simulink model "feedback_plant2"  (R2016a)
settings: Solver=FixedStepAuto  StartTime=0.0  StopTime=inf  MaxStep=0.1  RelTol=1e-3
libraries: xpcnilib x4, slrtlib x2
settings Model: ModifiedByFormat=The MathWorks Inc.  Creator=The MathWorks, Inc.  LastModifiedBy=The MathWorks Inc.
settings SolverCC: EnableConcurrentExecution=on
settings DataIOCC: LimitDataPoints=on  SaveFormat=Array  SaveOutput=off  SignalLogging=off  DSMLogging=off  SaveTime=off
settings OptimizationCC: BlockReduction=off  DefaultParameterBehavior=Inlined  OptimizeBlockIOStorage=off  BufferReuse=off  GlobalBufferReuse=off  ExpressionFolding=off  ExpressionDepthLimit=2147483647  LocalBlockOutputs=off
settings DebuggingCC: UnderspecifiedInitializationDetection=Classic  MergeDetectMultiDrivingBlocksExec=none  SolverPrmCheckMsg=warning  FcnCallInpInsideContextMsg=EnableAllAsWarning  AllowSymbolicDim=off  StateNameClashWarn=warning
settings HardwareCC: ProdBitPerPointer=32  ProdLargestAtomicFloat=None  ProdWordSize=32  ProdLongLongMode=on  ProdHWDeviceType=Generic->32-bit x86 compatible
settings ModelReferenceCC: ModelReferenceNumInstancesAllowed=Single  ModelReferenceMinAlgLoopOccurrences=on  PropagateSignalLabelsOutOfModel=off
settings RTWCC: SystemTargetFile=slrt.tlc  TemplateMakefile=slrt_default_tmf  Description=Simulink Real-Time
settings CodeAppCC: MaxIdLength=50
settings ConfigComp: CovModelRefEnable=Off  CovSFcnEnable=off

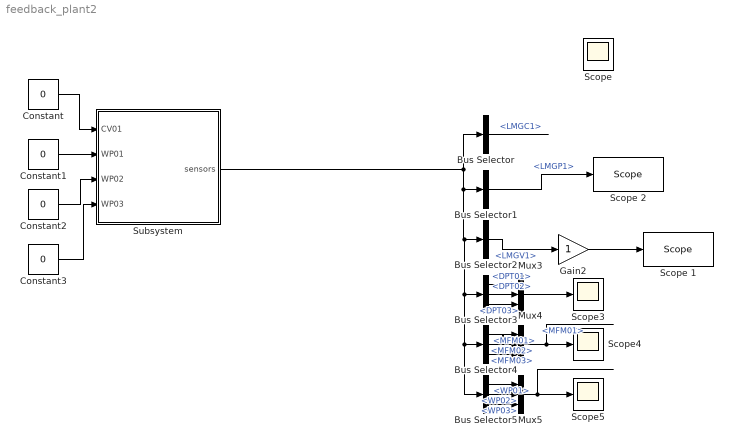
== system feedback_plant2 ==
  Bus Selector : BusSelector  OutputSignals=LMGC1
  Bus Selector1 : BusSelector  OutputSignals=LMGP1
  Bus Selector2 : BusSelector  OutputSignals=LMGV1
  Bus Selector3 : BusSelector  OutputSignals=DPT01,DPT02,DPT03
  Bus Selector4 : BusSelector  OutputSignals=MFM01,MFM02,MFM03
  Bus Selector5 : BusSelector  OutputSignals=WP01,WP02,WP03
  Constant{,1..3} (4 alike) : Constant  Value=0
  Gain2 : Gain
  Mux3 : Mux  Inputs=3
  Mux4 : Mux  Inputs=3
  Mux5 : Mux  Inputs=3
  Scope{,3..5} (4 alike) : Scope
  Scope 1 : slrtlib/Displays and Logging/Scope   scopeno=1  scopetype=Target  autostart=on  viewmode=Numerical  formatstr='%15.6f'  grid=on  ylimits=[0,0]  nosamples=250  noprepostsamples=0  interleave=1  triggermode=FreeRun  triggersignal=1  trigsignalfromport=off  triggerlevel=0.0  triggerslope=Either  triggerscope=1  triggersample=0  filename=data.dat  mode=Lazy  writesize=512  autorestart=off  dynamicfilemode=off  maxwritefilesize=512*1024^2
  Scope 2 : slrtlib/Displays and Logging/Scope   scopeno=2  scopetype=Target  autostart=on  viewmode=Numerical  formatstr='%15.6f'  grid=on  ylimits=[0,0]  nosamples=250  noprepostsamples=0  interleave=1  triggermode=FreeRun  triggersignal=1  trigsignalfromport=off  triggerlevel=0.0  triggerslope=Either  triggerscope=1  triggersample=0  filename=data.dat  mode=Lazy  writesize=512  autorestart=off  dynamicfilemode=off  maxwritefilesize=512*1024^2
  Subsystem : Subsystem
  wires:
  Mux3/1 -> Scope3/1
  Mux4/1 -> Scope4/1  "<MFM01>"
  Mux5/1 -> Scope5/1
  Constant/1 -> Subsystem/1(CV01)
  Constant1/1 -> Subsystem/2(WP01)
  Constant2/1 -> Subsystem/3(WP02)
  Constant3/1 -> Subsystem/4(WP03)
  Bus Selector3/1 -> Mux3/1  "<DPT01>"
  Bus Selector3/3 -> Mux3/3  "<DPT03>"
  Bus Selector3/2 -> Mux3/2  "<DPT02>"
  Bus Selector4/1 -> Mux4/1  "<MFM01>"
  Bus Selector4/3 -> Mux4/3  "<MFM03>"
  Bus Selector4/2 -> Mux4/2  "<MFM02>"
  Bus Selector5/1 -> Mux5/1  "<WP01>"
  Bus Selector5/2 -> Mux5/2  "<WP02>"
  Bus Selector5/3 -> Mux5/3  "<WP03>"
  Bus Selector/1 -> ?  "<LMGC1>"
  Subsystem/1(sensors) -> Bus Selector/1, Bus Selector5/1, Bus Selector4/1, Bus Selector3/1, Bus Selector2/1, Bus Selector1/1
  Bus Selector1/1 -> Scope 2/1  "<LMGP1>"
  Gain2/1 -> Scope 1/1
  Bus Selector2/1 -> Gain2/1  "<LMGV1>"

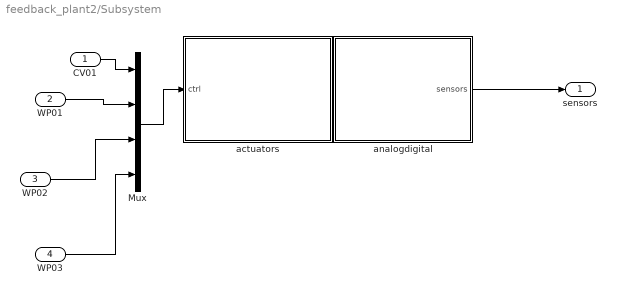
== system feedback_plant2/Subsystem ==
  CV01 : Inport
  WP01 : Inport  Port=2
  WP02 : Inport  Port=3
  WP03 : Inport  Port=4
  Mux : Mux
  actuators : Subsystem  mask{actuators_list={'CV03', 'CV05'}, subsystem=[3,1]}
      mask init:
      | %%Get analog channels
      | actuators = evalin('base','actuators');
      | 
      | subsystem = sprintf('[%d,%d]', subsystem(1), subsystem(2));
      | 
      | %actuators = actuators(strcmp(subsystem,{actuators.PCIslot}));
      | 
      | src_block = find_system(gcb, 'LookUnderMasks', 'on','Name', 'DA_sink');
      | maskObj = Simulink.Mask.get(src_block{1});
      | 
      | if(isempty(actuators))
      |    error('There are no analog outputs in the given card'); 
      | end
      | 
      | maskObj.Parameters(1,5).Value = subsystem;
      | maskObj.Parameters(1,1).Value = mat2str([actuators.Channel]+1);
      | Simulink.Block.eval(src_block{1});
      | 
      | %Find block
      | transform_blk = find_system(gcb, 'LookUnderMasks', 'on','Name', 'transform');
      | 
      | outputnames = {actuators.Name};
      | outputs = strjoin(outputnames,',');
      | 
      | sigcount = numel(outputnames);
      | sigstring = num2str(sigcount);
      | 
      | %Transform block
      | transform_blk = find_system(gcb, 'LookUnderMasks', 'on','Name', 'transform');
      | lines{1}=['function [' outputs ']  = fcn(u,gain,offset)'];
      | lines{2}='   y = u.*gain-offset;';
      | for i=1:numel(outputnames)
      |    %start at 4
      |    lines{2+i} = [ outputnames{i} ' = y(' num2str(i) ');'];
      | end
      | outputscript = strjoin(lines,'\n');
      | matlabfunctionfromstring(transform_blk{1}, outputscript);
      | Simulink.Block.eval(transform_blk{1});
      | 
      | %Delete lines
      | connections = find_system(gcb,'findall','on','LookUnderMasks', 'on','SearchDepth', 1,'type','line');
      | delete_line(connections);
      | 
      | for i=1:numel(outputnames)
      |    add_line(gcb,['transform/' num2str(i) ],['DA_sink/' num2str(i)],'autorouting','on');
      | end
      | 
      | %Transform block
      | add_line(gcb,'ctrl/1','transform/1','autorouting','on')
      | add_line(gcb,'gain/1','transform/2','autorouting','on')
      | add_line(gcb,'offset/1','transform/3','autorouting','on')
      | 
      | gain = [actuators.Gain]';
      | offset = [actuators.Offset]';
  analogdigital : Subsystem
      mask init:
      | block = find_system(gcb, 'SearchDepth',1, 'LookUnderMasks', 'on', 'FollowLinks', 'on', 'FunctionName', 'adnipcim');
      | sensors = evalin('base', 'sensors');
      | 
      | % Split by sensors card
      | C = unique({sensors.PCIslot});
      | % Should be same amount of internal blocks
      | assert(numel(C) == numel(block), 'There are the wrong number of input cards vs internal blocks')
      | 
      | %Delete lines
      | connections = find_system(gcb,'findall','on','LookUnderMasks', 'on','SearchDepth', 1,'type','line');
      | delete_line(connections);
      | 
      | Simulink.Block.eval([gcb '/collector']);
      | 
      | %% Find and connect sensors for each card
      | for i = 1:numel(block)
      |     % Split block to get card name
      |     D = strsplit(block{i},'/');
      |     card = D{end};
      |     
      |     block_specific = block{i};
      |     
      |     % Find corrosponding sensors
      |     signals_indices = find(cellfun(@(x)isequal(x,card), {sensors.PCIslot}));
      |     
      |     % Create lines
      |     for k = 1:numel(signals_indices)  
      |         from_port = [card '/', num2str(sensors(signals_indices(k)).Channel+1)];
      |         to_port = ['collector/', num2str(signals_indices(k))];
      | 
      |         add_line(gcb, from_port, to_port, 'autorouting','on');
      |     end
      | end
      | 
      | gain = [sensors.Gain];
      | offset = [sensors.Offset];
      | 
      | add_line(gcb, 'collector/1', 'conversion/1', 'autorouting','on')
      | add_line(gcb, 'conversion/1', 'sigcon/1', 'autorouting','on')
      | add_line(gcb, 'sigcon/1', 'sensors/1', 'autorouting','on')
      | 
      | % For internal use to assign values to bus
      | structFromBus = Simulink.Bus.createMATLABStruct('sensors_bus');
  sensors : Outport
  wires:
  WP01/1 -> Mux/2
  WP02/1 -> Mux/3
  CV01/1 -> Mux/1
  Mux/1 -> actuators/1(ctrl)
  WP03/1 -> Mux/4
  analogdigital/1(sensors) -> sensors/1

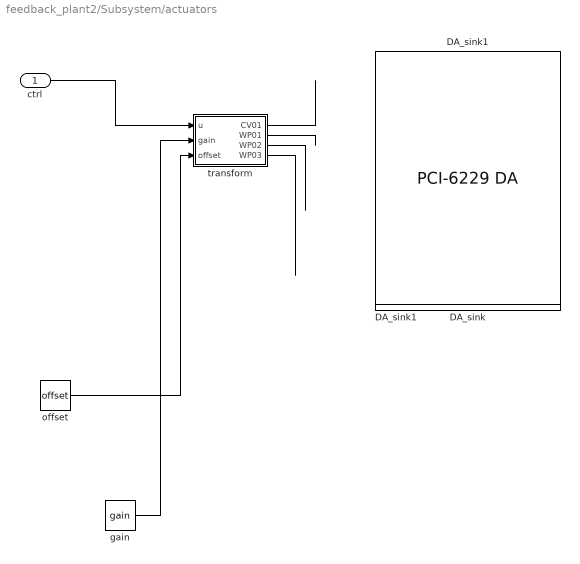
== system feedback_plant2/Subsystem/actuators ==
  ctrl : Inport
  DA_sink : xpcnilib/D//A/M Series/PCI-6229 DA  channel=[4 1 2 3]  reset=[1]  initValue=[0]  sampletime=T_sample_control  slot=[3,1]
  DA_sink1 : xpcnilib/D//A/M Series/PCI-6229 DA  channel=[4 1 2 3]  reset=[1]  initValue=[0]  sampletime=T_sample_control  slot=[3,1]
  DA_sink1 : xpcnilib/D//A/M Series/PCI-6229 DA  channel=[4 1 2 3]  reset=[1]  initValue=[0]  sampletime=T_sample_control  slot=[3,1]
  gain : Constant  Value=gain
  offset : Constant  Value=offset
  transform : MATLAB Function  TreatAsAtomicUnit=on
  wires:
  transform/1(CV01) -> ?
  transform/2(WP01) -> ?
  transform/3(WP02) -> ?
  transform/4(WP03) -> ?
  ctrl/1 -> transform/1(u)
  gain/1 -> transform/2(gain)
  offset/1 -> transform/3(offset)

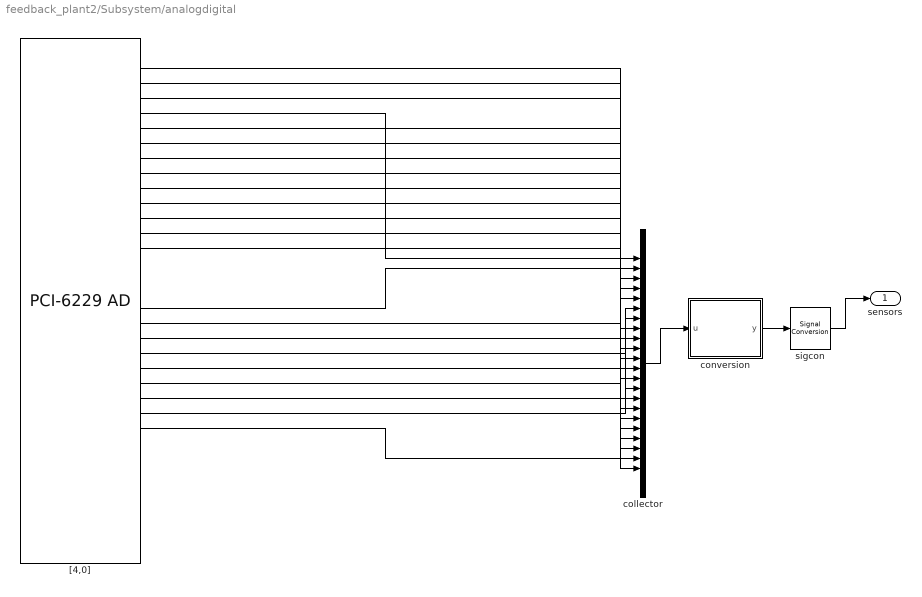
== system feedback_plant2/Subsystem/analogdigital ==
  "[4,0]" : xpcnilib/A//D/M Series/PCI-6229 AD  channel=[1 2 3 4 5 6 7 8 9 10 11 12 13 14 15 16 17 18 19 20 21 22 23 24 25 26 27 28 29 30 31 32]  range=[10]  coupling=[0]  scantime=5e-6  sampletime=T_sample_control  slot=[3,1]
  collector : Mux  Inputs=numel(sensors)
  conversion : MATLAB Function  TreatAsAtomicUnit=on
  sigcon : SignalConversion  ConversionOutput=Nonvirtual bus  OverrideOpt=off
  sensors : Outport
  wires:
  "[4,0]"/4 -> collector/1
  "[4,0]"/17 -> collector/2
  "[4,0]"/5 -> collector/3
  "[4,0]"/11 -> collector/4
  "[4,0]"/8 -> collector/5
  "[4,0]"/20 -> collector/6
  "[4,0]"/23 -> collector/7
  "[4,0]"/1 -> collector/8
  "[4,0]"/18 -> collector/9
  "[4,0]"/6 -> collector/10
  "[4,0]"/12 -> collector/11
  "[4,0]"/9 -> collector/12
  "[4,0]"/21 -> collector/13
  "[4,0]"/24 -> collector/14
  "[4,0]"/2 -> collector/15
  "[4,0]"/19 -> collector/16
  "[4,0]"/7 -> collector/17
  "[4,0]"/13 -> collector/18
  "[4,0]"/10 -> collector/19
  "[4,0]"/22 -> collector/20
  "[4,0]"/25 -> collector/21
  "[4,0]"/3 -> collector/22
  collector/1 -> conversion/1(u)
  conversion/1(y) -> sigcon/1
  sigcon/1 -> sensors/1

== matlab function feedback_plant2/Subsystem/actuators/transform ==
  data: u input; CV01 output; gain input; offset input; WP01 output; WP02 output; WP03 output
function [CV01,WP01,WP02,WP03]  = fcn(u,gain,offset)
   y = u.*gain-offset;
CV01 = y(1);
WP01 = y(2);
WP02 = y(3);
WP03 = y(4);

== matlab function feedback_plant2/Subsystem/analogdigital/conversion ==
  data: u input; y output Bus: sensors_bus size=1; gain parameter; offset parameter; structFromBus parameter
function y = fcn(u, gain, offset, structFromBus)
u = u +5;
final = gain.*u.'-offset;

SNames = fieldnames(structFromBus); 
for loopIndex = 1:numel(SNames) 
    structFromBus.(SNames{loopIndex}) = final(loopIndex);
end

y = structFromBus;

end
